simulink model "gm_rmsNormalization"  (R2025a)
settings: Solver=FixedStepDiscrete  StartTime=0.0  StopTime=simStopTime  FixedStep=1  RelTol=1e-3
libraries: simulink x23
(part 2 of 3)

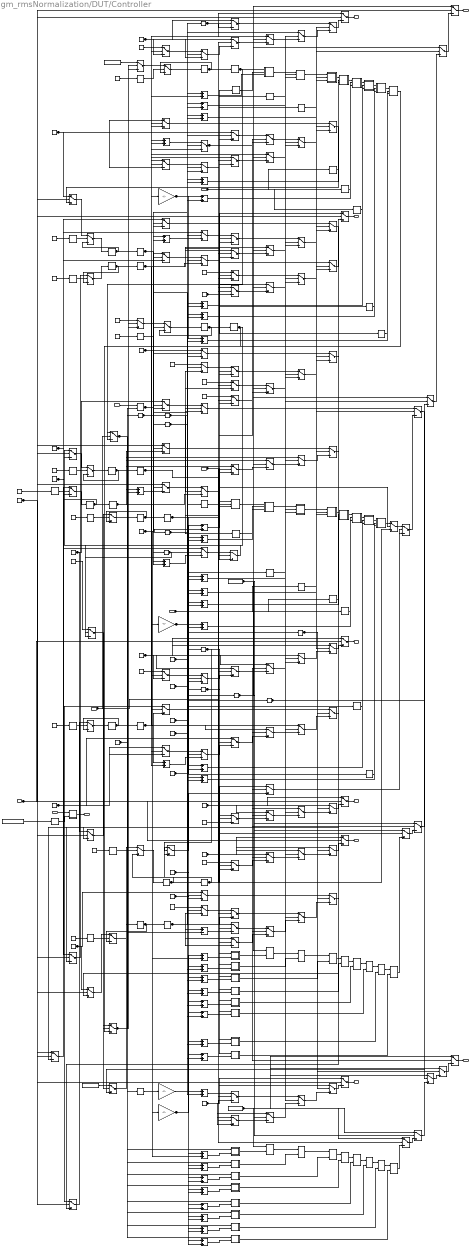
== system gm_rmsNormalization/DUT/Controller ==
  reset : Inport  OutDataTypeStr=boolean  PortDimensions=1  SampleTime=1
  start : Inport  Port=2  OutDataTypeStr=boolean  PortDimensions=1  SampleTime=1
  cfgGammaBeat : Inport  Port=3  OutDataTypeStr=single  PortDimensions=[1 8]  SampleTime=1
  cfgGammaValid : Inport  Port=4  OutDataTypeStr=boolean  PortDimensions=1  SampleTime=1
  ddrDataBeat : Inport  Port=5  OutDataTypeStr=single  PortDimensions=[1 8]  SampleTime=1
  ddrDataValid : Inport  Port=6  OutDataTypeStr=boolean  PortDimensions=1  SampleTime=1
  currentSumIn : Inport  Port=7  OutDataTypeStr=single  PortDimensions=1  SampleTime=1
  Assignment : Assignment  IndexOptions=Index vector (dialog)  Indices=double(8)  OutputSizes=double(0)
  Assignment1 : Assignment  IndexOptions=Index vector (dialog)  Indices=double(8)  OutputSizes=double(0)
  Assignment10 : Assignment  IndexOptions=Index vector (dialog)  Indices=double(3)  OutputSizes=double(0)
  Assignment11 : Assignment  IndexOptions=Index vector (dialog)  Indices=double(3)  OutputSizes=double(0)
  Assignment12 : Assignment  IndexOptions=Index vector (dialog)  Indices=double(2)  OutputSizes=double(0)
  Assignment13 : Assignment  IndexOptions=Index vector (dialog)  Indices=double(2)  OutputSizes=double(0)
  Assignment14 : Assignment  IndexOptions=Index vector (dialog)  Indices=double(1)  OutputSizes=double(0)
  Assignment15 : Assignment  IndexOptions=Index vector (dialog)  Indices=double(1)  OutputSizes=double(0)
  Assignment16 : Subsystem
  Assignment17 : Subsystem
  Assignment18 : Subsystem
  Assignment19 : Subsystem
  Assignment2 : Assignment  IndexOptions=Index vector (dialog)  Indices=double(7)  OutputSizes=double(0)
  Assignment20 : Subsystem
  Assignment21 : Subsystem
  Assignment22 : Subsystem
  Assignment23 : Subsystem
  Assignment24 : Subsystem
  Assignment25 : Subsystem
  Assignment26 : Subsystem
  Assignment27 : Subsystem
  Assignment28 : Subsystem
  Assignment29 : Subsystem
  Assignment3 : Assignment  IndexOptions=Index vector (dialog)  Indices=double(7)  OutputSizes=double(0)
  Assignment30 : Subsystem
  Assignment31 : Subsystem
  Assignment4 : Assignment  IndexOptions=Index vector (dialog)  Indices=double(6)  OutputSizes=double(0)
  Assignment5 : Assignment  IndexOptions=Index vector (dialog)  Indices=double(6)  OutputSizes=double(0)
  Assignment6 : Assignment  IndexOptions=Index vector (dialog)  Indices=double(5)  OutputSizes=double(0)
  Assignment7 : Assignment  IndexOptions=Index vector (dialog)  Indices=double(5)  OutputSizes=double(0)
  Assignment8 : Assignment  IndexOptions=Index vector (dialog)  Indices=double(4)  OutputSizes=double(0)
  Assignment9 : Assignment  IndexOptions=Index vector (dialog)  Indices=double(4)  OutputSizes=double(0)
  Selector : Subsystem
  Selector1 : Subsystem
  Selector10 : Selector  InputPortWidth=8  IndexOptions=Index vector (dialog)  Indices=double(7)  OutputSizes=double(0)
  Selector11 : Subsystem
  Selector12 : Subsystem
  Selector13 : Selector  InputPortWidth=8  IndexOptions=Index vector (dialog)  Indices=double(6)  OutputSizes=double(0)
  Selector14 : Subsystem
  Selector15 : Subsystem
  Selector16 : Selector  InputPortWidth=8  IndexOptions=Index vector (dialog)  Indices=double(5)  OutputSizes=double(0)
  Selector17 : Subsystem
  Selector18 : Subsystem
  Selector19 : Selector  InputPortWidth=8  IndexOptions=Index vector (dialog)  Indices=double(4)  OutputSizes=double(0)
  Selector2 : Subsystem
  Selector20 : Subsystem
  Selector21 : Selector  InputPortWidth=8  IndexOptions=Index vector (dialog)  Indices=double(8)  OutputSizes=double(0)
  Selector22 : Selector  InputPortWidth=8  IndexOptions=Index vector (dialog)  Indices=double(3)  OutputSizes=double(0)
  Selector23 : Selector  InputPortWidth=8  IndexOptions=Index vector (dialog)  Indices=double(7)  OutputSizes=double(0)
  Selector24 : Selector  InputPortWidth=8  IndexOptions=Index vector (dialog)  Indices=double(2)  OutputSizes=double(0)
  Selector25 : Selector  InputPortWidth=8  IndexOptions=Index vector (dialog)  Indices=double(6)  OutputSizes=double(0)
  Selector26 : Selector  InputPortWidth=8  IndexOptions=Index vector (dialog)  Indices=double(1)  OutputSizes=double(0)
  Selector27 : Selector  InputPortWidth=8  IndexOptions=Index vector (dialog)  Indices=double(5)  OutputSizes=double(0)
  Selector28 : Selector  InputPortWidth=8  IndexOptions=Index vector (dialog)  Indices=double(4)  OutputSizes=double(0)
  Selector29 : Selector  InputPortWidth=8  IndexOptions=Index vector (dialog)  Indices=double(3)  OutputSizes=double(0)
  Selector3 : Subsystem
  Selector30 : Selector  InputPortWidth=8  IndexOptions=Index vector (dialog)  Indices=double(2)  OutputSizes=double(0)
  Selector31 : Selector  InputPortWidth=8  IndexOptions=Index vector (dialog)  Indices=double(1)  OutputSizes=double(0)
  Selector4 : Subsystem
  Selector5 : Subsystem
  Selector6 : Subsystem
  Selector7 : Selector  InputPortWidth=8  IndexOptions=Index vector (dialog)  Indices=double(8)  OutputSizes=double(0)
  Selector8 : Subsystem
  Selector9 : Subsystem
  adder{,1..32,34..35,37..38} (37 alike) : Sum  OutDataTypeStr=uint16  AccumDataTypeStr=uint16  RndMeth=Nearest  SaturateOnIntegerOverflow=on  SampleTime=1
  adder33 : Subsystem
      mask Display: disp('NFP\nadd');
  adder36 : Sum  OutDataTypeStr=uint8  AccumDataTypeStr=uint8  RndMeth=Nearest  SaturateOnIntegerOverflow=on  SampleTime=1
  and : Logic  AllPortsSameDT=off  OutDataTypeStr=boolean  SampleTime=1
  compare : simulink/Logic and Bit Operations/Compare To Constant  relop=~=  const=0  OutDataTypeStr=boolean
  compare1 : simulink/Logic and Bit Operations/Compare To Constant  relop===  const=191  OutDataTypeStr=boolean
  compare10 : simulink/Logic and Bit Operations/Compare To Constant  relop=<  const=192  OutDataTypeStr=boolean
  compare2 : simulink/Logic and Bit Operations/Compare To Constant  relop===  const=63  OutDataTypeStr=boolean
  compare3 : simulink/Logic and Bit Operations/Compare To Constant  relop===  const=3  OutDataTypeStr=boolean
  compare4 : simulink/Logic and Bit Operations/Compare To Constant  relop===  const=1  OutDataTypeStr=boolean
  compare5 : simulink/Logic and Bit Operations/Compare To Constant  relop===  const=191  OutDataTypeStr=boolean
  compare6 : simulink/Logic and Bit Operations/Compare To Constant  relop===  const=0  OutDataTypeStr=boolean
  compare7 : simulink/Logic and Bit Operations/Compare To Constant  relop===  const=191  OutDataTypeStr=boolean
  compare8 : simulink/Logic and Bit Operations/Compare To Constant  relop===  const=2  OutDataTypeStr=boolean
  compare9 : simulink/Logic and Bit Operations/Compare To Constant  relop===  const=0  OutDataTypeStr=boolean
  const : Constant  Value=single(0.0015360000543296337)  VectorParams1D=off  OutDataTypeStr=single  SampleTime=1
  const1 : Constant  Value="repmat(single(0),[1  8])"  VectorParams1D=off  OutDataTypeStr=single  SampleTime=1
  const{8..11,13..14} (6 alike) : Constant  VectorParams1D=off  OutDataTypeStr=boolean  SampleTime=1
  const12 : Constant  Value=0  VectorParams1D=off  OutDataTypeStr=uint8  SampleTime=1
  const{3..4,6..7,15,19} (6 alike) : Constant  Value=0  VectorParams1D=off  OutDataTypeStr=boolean  SampleTime=1
  const16 : Constant  VectorParams1D=off  OutDataTypeStr=uint8  SampleTime=1
  const17 : Constant  Value=8  VectorParams1D=off  OutDataTypeStr=uint16  SampleTime=1
  const{5,18,27..28,35} (5 alike) : Constant  Value=0  VectorParams1D=off  OutDataTypeStr=uint16  SampleTime=1
  const2 : Constant  Value="repmat(single(0),[1  8])"  VectorParams1D=off  OutDataTypeStr=single  SampleTime=1
  const20 : Constant  Value=7  VectorParams1D=off  OutDataTypeStr=uint16  SampleTime=1
  const21 : Constant  Value=4  VectorParams1D=off  OutDataTypeStr=uint8  SampleTime=1
  const22 : Constant  Value=3  VectorParams1D=off  OutDataTypeStr=uint8  SampleTime=1
  const23 : Constant  Value=2  VectorParams1D=off  OutDataTypeStr=uint8  SampleTime=1
  const24 : Constant  Value="repmat(single(0),[1  1536])"  VectorParams1D=off  OutDataTypeStr=single  SampleTime=1
  const25 : Constant  Value=6  VectorParams1D=off  OutDataTypeStr=uint16  SampleTime=1
  const26 : Constant  Value=0  VectorParams1D=off  OutDataTypeStr=uint8  SampleTime=1
  const29 : Constant  Value=5  VectorParams1D=off  OutDataTypeStr=uint16  SampleTime=1
  const30 : Constant  Value="repmat(single(0),[1  1536])"  VectorParams1D=off  OutDataTypeStr=single  SampleTime=1
  const31 : Constant  Value=4  VectorParams1D=off  OutDataTypeStr=uint16  SampleTime=1
  const32 : Constant  Value=3  VectorParams1D=off  OutDataTypeStr=uint16  SampleTime=1
  const33 : Constant  VectorParams1D=off  OutDataTypeStr=uint16  SampleTime=1
  const34 : Constant  Value=0  VectorParams1D=off  OutDataTypeStr=uint8  SampleTime=1
  const36 : Constant  Value=2  VectorParams1D=off  OutDataTypeStr=uint16  SampleTime=1
  const37 : Constant  VectorParams1D=off  OutDataTypeStr=uint8  SampleTime=1
  const38 : Constant  Value=22  VectorParams1D=off  OutDataTypeStr=uint8  SampleTime=1
  delayMatch : Delay  DelayLength=double(70)  InitialCondition=0  SampleTime=1
  delayMatch{1..10} (10 alike) : Delay  DelayLength=double(41)  InitialCondition=0  SampleTime=1
  dtc : DataTypeConversion  OutDataTypeStr=uint16  RndMeth=Nearest  SampleTime=1
  gain : Gain  Gain="fi(0,0,16,0,\"hex\",\"00c0\")"  ParamDataTypeStr=fixdt(0, 16, 0)  OutDataTypeStr=uint16  RndMeth=Nearest  SaturateOnIntegerOverflow=on  SampleTime=1
  gain1 : Gain  Gain="fi(0,0,16,0,\"hex\",\"0008\")"  ParamDataTypeStr=fixdt(0, 16, 0)  OutDataTypeStr=uint16  RndMeth=Nearest  SaturateOnIntegerOverflow=on  SampleTime=1
  gain2 : Gain  Gain="fi(0,0,16,0,\"hex\",\"0008\")"  ParamDataTypeStr=fixdt(0, 16, 0)  OutDataTypeStr=uint16  RndMeth=Nearest  SaturateOnIntegerOverflow=on  SampleTime=1
  gain3 : Gain  Gain="fi(0,0,16,0,\"hex\",\"0008\")"  ParamDataTypeStr=fixdt(0, 16, 0)  OutDataTypeStr=uint16  RndMeth=Nearest  SaturateOnIntegerOverflow=on  SampleTime=1
  intdelay{,1..9} (10 alike) : Delay  DelayLength=double(1)  InitialCondition=0  SampleTime=1
  intdelay_enbsw{,4,6,9} (4 alike) : Switch  Criteria=u2 ~= 0  Threshold=double(0)  OutDataTypeStr=uint16  SampleTime=1  SaturateOnIntegerOverflow=off  InputSameDT=off
  intdelay_enbsw1 : Switch  Criteria=u2 ~= 0  Threshold=double(0)  OutDataTypeStr=boolean  SampleTime=1  SaturateOnIntegerOverflow=off  InputSameDT=off
  intdelay_enbsw2 : Switch  Criteria=u2 ~= 0  Threshold=double(0)  OutDataTypeStr=uint8  SampleTime=1  SaturateOnIntegerOverflow=off  InputSameDT=off
  intdelay_enbsw3 : Switch  Criteria=u2 ~= 0  Threshold=double(0)  OutDataTypeStr=uint8  SampleTime=1  SaturateOnIntegerOverflow=off  InputSameDT=off
  intdelay_enbsw5 : Switch  Criteria=u2 ~= 0  Threshold=double(0)  OutDataTypeStr=uint8  SampleTime=1  SaturateOnIntegerOverflow=off  InputSameDT=off
  intdelay_enbsw7 : Switch  Criteria=u2 ~= 0  Threshold=double(0)  OutDataTypeStr=single  SampleTime=1  SaturateOnIntegerOverflow=off  InputSameDT=off
  intdelay_enbsw8 : Switch  Criteria=u2 ~= 0  Threshold=double(0)  OutDataTypeStr=single  SampleTime=1  SaturateOnIntegerOverflow=off  InputSameDT=off
  sigspec{,2,5,9} (4 alike) : SignalSpecification  OutDataTypeStr=uint16  Dimensions=1
  sigspec1 : SignalSpecification  OutDataTypeStr=boolean  Dimensions=1
  sigspec3 : SignalSpecification  OutDataTypeStr=uint8  Dimensions=1
  sigspec4 : SignalSpecification  OutDataTypeStr=uint8  Dimensions=1
  sigspec6 : SignalSpecification  OutDataTypeStr=uint8  Dimensions=1
  sigspec7 : SignalSpecification  OutDataTypeStr=single  Dimensions=[1, 1536]
  sigspec8 : SignalSpecification  OutDataTypeStr=single  Dimensions=[1, 1536]
  stateControl{,1..9} (10 alike) : Constant  OutDataTypeStr=boolean  SampleTime=1
  subtract : Sum  Inputs=+-  OutDataTypeStr=uint8  AccumDataTypeStr=uint8  RndMeth=Nearest  SaturateOnIntegerOverflow=on  SampleTime=1
  switch{,1,8..9,16..17,25..26,35..36,99..106} (18 alike) : Switch  Criteria=u2 ~= 0  Threshold="fi(0,0,1,0,\"hex\",\"0\")"  OutDataTypeStr=single  SampleTime=1  SaturateOnIntegerOverflow=off  InputSameDT=off
  switch{2..3,5..7,10..11,13..15,18..19,21..24,27..28,31..34,37..38,40..46,50..52} (34 alike) : Switch  Criteria=u2 ~= 0  Threshold="fi(0,0,1,0,\"hex\",\"0\")"  OutDataTypeStr=boolean  SampleTime=1  SaturateOnIntegerOverflow=off  InputSameDT=off
  switch{4,12,20,29..30,39,47..49,53..58,74,82..90,97..98,107..117} (38 alike) : Switch  Criteria=u2 ~= 0  Threshold="fi(0,0,1,0,\"hex\",\"0\")"  OutDataTypeStr=uint16  SampleTime=1  SaturateOnIntegerOverflow=off  InputSameDT=off
  switch{59..73,75..81,91..96} (28 alike) : Switch  Criteria=u2 ~= 0  Threshold="fi(0,0,1,0,\"hex\",\"0\")"  OutDataTypeStr=uint8  SampleTime=1  SaturateOnIntegerOverflow=off  InputSameDT=off
  rsqrtOperand : Outport  SampleTime=1
  xBeatOut : Outport  Port=2  SampleTime=1
  gBeatOut : Outport  Port=3  SampleTime=1
  captureInvRms : Outport  Port=4  SampleTime=1
  outValid : Outport  Port=5  SampleTime=1
  ddrReadAddr : Outport  Port=6  SampleTime=1
  ddrReadEn : Outport  Port=7  SampleTime=1
  done : Outport  Port=8  SampleTime=1
  busy : Outport  Port=9  SampleTime=1
  wires:
  switch31/1 -> switch21/3
  intdelay_enbsw8/1 -> intdelay8/1
  const15/1 -> switch46/1
  Assignment26/1(Out1) -> Assignment27/1(In1)
  Assignment29/1(Out1) -> Assignment30/1(In1)
  Assignment1/1 -> switch36/3
  switch41/1 -> switch33/3
  switch34/1 -> switch23/3
  switch9/1 -> switch1/3
  Selector29/1 -> Assignment18/2(In2)
  switch104/1 -> intdelay_enbsw7/1
  Assignment24/1(Out1) -> Assignment25/1(In1)
  const30/1 -> switch105/1
  adder26/1 -> Assignment21/3(In3)
  Assignment13/1 -> Assignment11/1
  Assignment8/1 -> Assignment6/1
  Assignment21/1(Out1) -> Assignment22/1(In1)
  switch52/1 -> switch51/1
  switch39/1 -> switch29/3
  switch66/1 -> switch67/1
  switch14/1 -> switch6/3
  Selector4/1(Out1) -> Assignment4/2
  switch42/1 -> switch34/3
  switch25/1 -> switch16/3
  switch27/1 -> switch18/3
  switch10/1 -> switch2/3
  delayMatch10/1 -> intdelay_enbsw4/2
  switch12/1 -> switch4/3
  switch46/1 -> switch44/1
  Selector30/1 -> Assignment17/2(In2)
  adder2/1 -> Selector1/2(In2)
  switch15/1 -> switch7/3
  switch22/1 -> switch14/3
  switch60/1 -> switch61/3
  const10/1 -> switch37/1
  Assignment7/1 -> Assignment5/1
  const19/1 -> switch50/1
  compare6/1 -> switch65/2, switch72/2
  switch18/1 -> switch10/3
  const9/1 -> switch32/1
  adder25/1 -> Assignment25/3(In3)
  Assignment10/1 -> Assignment8/1
  adder10/1 -> Selector8/2(In2)
  switch72/1 -> switch62/1
  Assignment11/1 -> Assignment9/1
  switch65/1 -> switch64/1
  delayMatch6/1 -> intdelay_enbsw6/2
  switch101/1 -> switch102/1
  adder14/1 -> Selector12/2(In2)
  switch1/1 -> gBeatOut/1
  switch53/1 -> switch55/3
  switch51/1 -> switch50/3, and/2
  const23/1 -> switch91/1
  const36/1 -> adder25/2, adder31/2, adder17/2, adder19/2
  adder38/1 -> switch111/1
  switch28/1 -> switch19/3
  switch33/1 -> switch22/3
  delayMatch2/1 -> intdelay_enbsw9/2
  Selector26/1 -> Assignment24/2(In2)
  compare2/1 -> switch82/2, switch107/2, switch45/2, switch59/2, switch46/2, switch54/2, switch75/2
  currentSumIn/1 -> adder33/1(In1)
  switch87/1 -> switch89/3
  Selector19/1 -> Assignment27/2(In2)
  sigspec/1 -> gain2/1, compare1/1, adder34/1, switch48/3
  switch85/1 -> switch86/1
  switch40/1 -> switch31/3
  gain1/1 -> adder13/1, adder7/1, adder1/1, adder8/1, adder11/1, adder4/1, adder3/1, adder21/1, adder10/1, adder16/1, adder19/1, adder5/1, adder14/1, adder17/1, adder23/1, adder2/1
  switch23/1 -> switch15/3
  sigspec1/1 -> switch52/3, switch51/3
  const35/1 -> switch90/1, switch85/1, switch82/3, switch88/1
  switch113/1 -> switch114/1
  intdelay_enbsw1/1 -> intdelay1/1
  switch/1 -> xBeatOut/1
  stateControl3/1 -> delayMatch4/1
  compare9/1 -> switch115/2, switch12/2, switch15/2, switch13/2, switch11/2, switch89/2, switch58/2, switch79/2, switch10/2, switch69/2, switch14/2, switch94/2, switch8/2, switch103/2, switch9/2
  Assignment17/1(Out1) -> Assignment18/1(In1)
  const29/1 -> adder28/2, adder8/2, adder15/2, adder10/2
  const20/1 -> adder3/2, adder4/2, adder9/2, adder24/2
  switch24/1 -> switch15/1
  switch74/1 -> switch83/3
  Assignment/1 -> switch35/3
  Selector9/1(Out1) -> Assignment8/2
  switch77/1 -> switch78/3
  adder13/1 -> Selector11/2(In2)
  const/1 -> delayMatch/1
  Selector3/1(Out1) -> Assignment3/2
  adder6/1 -> Assignment31/3(In3)
  adder31/1 -> Assignment17/3(In3)
  switch88/1 -> switch89/1
  sigspec2/1 -> gain1/1, compare7/1, adder35/1, switch97/3, switch57/1, switch56/1
  stateControl7/1 -> delayMatch8/1
  adder15/1 -> Assignment28/3(In3)
  const37/1 -> adder36/2, subtract/2
  const17/1 -> adder2/2, adder6/2, adder1/2, adder20/2
  switch70/1 -> switch69/1
  switch83/1 -> switch84/3
  const5/1 -> switch39/1, switch39/3, switch4/1, switch30/3, switch29/1, switch12/1
  Selector12/1(Out1) -> Assignment10/2
  Selector/1(Out1) -> Assignment/2
  adder20/1 -> Assignment23/3(In3)
  switch57/1 -> switch58/3
  stateControl1/1 -> delayMatch2/1
  cfgGammaValid/1 -> switch51/2, switch106/2, switch48/2
  intdelay_enbsw9/1 -> intdelay9/1
  compare10/1 -> switch111/2, switch32/2, switch30/2
  switch38/1 -> switch28/3
  compare1/1 -> switch47/2, switch52/2
  adder9/1 -> Assignment30/3(In3)
  Assignment12/1 -> Assignment10/1
  compare5/1 -> switch85/2, switch91/2, switch66/2, switch112/2
  compare7/1 -> switch44/2, switch53/2, switch43/2, switch108/2, switch60/2, switch73/2, switch74/2
  switch106/1 -> Selector11/1(In1), switch105/3, Selector5/1(In1), Selector1/1(In1), Selector14/1(In1), Selector20/1(In1), Selector8/1(In1), Selector17/1(In1), Selector3/1(In1)
  const26/1 -> switch81/1, switch80/1, switch75/1
  switch11/1 -> switch3/3
  intdelay2/1 -> sigspec3/1, intdelay_enbsw2/3
  switch78/1 -> switch79/3
  ddrDataBeat/1 -> Selector31/1, Selector27/1, Selector23/1, Selector28/1, Selector29/1, Selector30/1, Selector25/1, Selector21/1
  switch80/1 -> switch79/1
  stateControl6/1 -> delayMatch7/1
  intdelay4/1 -> sigspec5/1, intdelay_enbsw4/3
  Selector27/1 -> Assignment20/2(In2)
  sigspec3/1 -> compare6/1, subtract/1, switch70/3, switch66/3, switch63/3, switch63/1, switch65/1, switch67/3
  switch29/1 -> switch20/3
  Selector5/1(Out1) -> Assignment5/2
  switch108/1 -> switch109/3
  switch94/1 -> switch96/3
  const25/1 -> adder5/2, adder7/2, adder26/2, adder12/2
  switch116/1 -> switch115/1
  switch69/1 -> switch71/3
  const6/1 -> switch32/3, switch13/1, switch40/3, switch40/1, switch5/1, switch31/1
  Assignment31/1(Out1) -> switch106/1
  start/1 -> and/1
  sigspec5/1 -> gain3/1, switch82/1, switch88/3, adder37/1, compare5/1, switch83/1, switch74/3, switch86/3, switch84/1
  switch48/1 -> switch49/3
  switch84/1 -> switch87/3
  switch64/1 -> switch68/3
  gain3/1 -> adder30/1, adder26/1, adder31/1, adder20/1, adder24/1, adder28/1, adder29/1, adder32/1
  const7/1 -> switch14/1, switch45/3, switch22/1, switch43/3, switch33/1, switch41/1, switch6/1
  compare8/1 -> switch33/2, switch64/2, switch84/2, switch27/2, switch28/2, switch56/2, switch31/2, switch100/2, switch110/2, switch77/2, switch62/2, switch29/2, switch34/2, switch25/2, switch26/2
  switch4/1 -> ddrReadAddr/1
  adder7/1 -> Selector5/2(In2)
  switch99/1 -> switch100/3
  adder28/1 -> Assignment20/3(In3)
  Selector6/1(Out1) -> Assignment6/2
  sigspec7/1 -> Selector12/1(In1), Selector4/1(In1), Assignment16/1(In1), Selector18/1(In1), Selector/1(In1), Selector2/1(In1), Selector9/1(In1), Selector6/1(In1), Selector15/1(In1), switch103/1, switch100/1, switch101/3, switch99/1, switch99/3
  intdelay7/1 -> sigspec7/1, intdelay_enbsw7/3
  switch79/1 -> switch81/3
  switch98/1 -> intdelay_enbsw6/1
  adder30/1 -> Assignment18/3(In3)
  Selector23/1 -> Assignment22/2(In2)
  compare3/1 -> switch63/2, switch76/2, switch40/2, switch109/2, switch61/2, switch42/2, switch38/2, switch39/2, switch37/2, switch41/2, switch55/2, switch83/2, switch35/2, switch36/2, switch99/2
  adder29/1 -> Assignment19/3(In3)
  switch45/1 -> switch43/1
  switch86/1 -> switch87/1
  Assignment28/1(Out1) -> Assignment29/1(In1)
  intdelay1/1 -> sigspec1/1, intdelay_enbsw1/3
  intdelay/1 -> sigspec/1, intdelay_enbsw/3
  switch117/1 -> intdelay_enbsw9/1
  sigspec6/1 -> switch60/3, compare3/1, compare/1, switch91/3, switch95/3, compare4/1, compare8/1, switch92/3, switch72/3, compare9/1
  const21/1 -> switch61/1
  switch76/1 -> switch77/3
  switch58/1 -> switch98/3
  const4/1 -> switch38/1, switch11/1, switch3/1, switch28/1, switch19/1
  switch67/1 -> switch68/1
  stateControl2/1 -> delayMatch3/1
  adder19/1 -> Selector17/2(In2)
  compare4/1 -> switch93/2, switch23/2, switch57/2, switch21/2, switch78/2, switch87/2, switch22/2, switch114/2, switch68/2, switch18/2, switch19/2, switch20/2, switch16/2, switch102/2, switch17/2
  Selector8/1(Out1) -> Assignment7/2
  intdelay8/1 -> sigspec8/1, intdelay_enbsw8/3
  switch100/1 -> switch102/3
  Assignment6/1 -> Assignment4/1
  const16/1 -> switch59/3, switch95/1
  Selector31/1 -> Assignment16/2(In2)
  switch89/1 -> switch90/3
  switch16/1 -> switch8/3
  Selector11/1(Out1) -> Assignment9/2
  sigspec4/1 -> adder36/1, dtc/1, compare2/1, switch80/3, switch77/1, switch78/1, switch73/3, switch76/1
  intdelay_enbsw/1 -> intdelay/1
  sigspec9/1 -> switch108/3, switch116/3, compare10/1, adder38/1, switch107/1, adder/2, switch109/1, switch111/3, switch110/1
  switch47/1 -> switch48/1
  const8/1 -> switch46/3, switch34/1, switch24/1, switch44/3, switch42/1, switch23/1
  switch21/1 -> switch13/3
  switch112/1 -> switch113/1
  switch103/1 -> switch104/3
  ddrDataValid/1 -> switch86/2, switch92/2, switch67/2, switch101/2, switch113/2
  Selector25/1 -> Assignment21/2(In2)
  delayMatch/1 -> adder33/2(In2)
  const3/1 -> switch37/3, switch18/1, switch10/1, switch27/1, switch2/1
  Selector15/1(Out1) -> Assignment12/2
  const2/1 -> Assignment15/1, switch26/1, switch17/1, switch9/1, switch36/1, switch1/1
  const27/1 -> switch98/1, switch54/1, switch97/1, switch55/1, switch54/3
  intdelay9/1 -> sigspec9/1, intdelay_enbsw9/3
  compare/1 -> switch24/3, switch7/1
  adder/1 -> switch30/1
  Selector16/1 -> Assignment28/2(In2)
  intdelay_enbsw6/1 -> intdelay6/1
  adder33/1(Out1) -> rsqrtOperand/1
  Selector7/1 -> Assignment31/2(In2)
  const18/1 -> switch117/1, switch116/1, switch112/1, switch107/3
  Assignment27/1(Out1) -> Assignment28/1(In1)
  intdelay_enbsw2/1 -> intdelay2/1
  reset/1 -> switch81/2, switch71/2, switch4/2, switch6/2, switch5/2, switch105/2, switch104/2, switch90/2, switch50/2, switch1/2, switch/2, switch98/2, switch7/2, switch3/2, switch117/2, switch2/2, switch96/2, switch49/2
  Selector2/1(Out1) -> Assignment2/2
  Selector28/1 -> Assignment19/2(In2)
  intdelay3/1 -> intdelay_enbsw3/3, sigspec4/1
  switch96/1 -> intdelay_enbsw5/1
  adder37/1 -> switch85/3
  adder24/1 -> Assignment22/3(In3)
  Assignment23/1(Out1) -> switch101/1
  and/1 -> switch97/2, switch80/2, switch88/2, switch116/2, switch24/2, switch70/2, switch95/2
  Selector13/1 -> Assignment29/2(In2)
  intdelay_enbsw4/1 -> intdelay4/1
  const32/1 -> adder22/2, adder14/2, adder16/2, adder30/2
  const34/1 -> switch70/1, switch71/1
  switch92/1 -> switch93/1
  switch55/1 -> switch56/3
  intdelay5/1 -> sigspec6/1, intdelay_enbsw5/3
  switch111/1 -> switch112/3, switch113/3
  const1/1 -> Assignment14/1, switch8/1, switch35/1, switch16/1, switch25/1, switch/1
  stateControl/1 -> delayMatch1/1
  switch30/1 -> switch20/1
  switch6/1 -> done/1
  switch7/1 -> busy/1
  Assignment5/1 -> Assignment3/1
  adder16/1 -> Selector14/2(In2)
  intdelay_enbsw3/1 -> intdelay3/1
  stateControl9/1 -> delayMatch10/1
  const28/1 -> switch49/1, switch47/1
  switch73/1 -> switch76/3
  cfgGammaBeat/1 -> Selector26/1, Selector16/1, Selector24/1, Selector13/1, Selector7/1, Selector22/1, Selector19/1, Selector10/1
  adder21/1 -> Selector18/2(In2)
  switch37/1 -> switch27/3
  adder36/1 -> switch75/3
  switch2/1 -> captureInvRms/1
  switch36/1 -> switch26/3
  switch20/1 -> switch12/3
  Selector10/1 -> Assignment30/2(In2)
  intdelay_enbsw5/1 -> intdelay5/1
  Selector1/1(Out1) -> Assignment1/2
  switch82/1 -> switch74/1
  Selector24/1 -> Assignment25/2(In2)
  adder23/1 -> Selector20/2(In2)
  const11/1 -> switch38/3
  switch107/1 -> switch108/1
  switch59/1 -> switch60/1
  const38/1 -> switch66/1
  delayMatch3/1 -> intdelay_enbsw1/2
  switch50/1 -> intdelay_enbsw1/1
  switch75/1 -> switch73/1
  delayMatch7/1 -> intdelay_enbsw/2
  Assignment18/1(Out1) -> Assignment19/1(In1)
  Assignment3/1 -> Assignment1/1
  switch68/1 -> switch69/3
  gain2/1 -> adder9/1, adder18/1, adder12/1, adder22/1, adder6/1, adder25/1, adder27/1, adder15/1
  const24/1 -> switch104/1
  Assignment19/1(Out1) -> Assignment20/1(In1)
  const31/1 -> adder18/2, adder29/2, adder13/2, adder11/2
  stateControl5/1 -> delayMatch6/1
  delayMatch8/1 -> intdelay_enbsw8/2
  Assignment20/1(Out1) -> Assignment21/1(In1)
  switch35/1 -> switch25/3
  switch17/1 -> switch9/3
  Assignment15/1 -> Assignment13/1
  switch13/1 -> switch5/3
  switch26/1 -> switch17/3
  stateControl8/1 -> delayMatch9/1
  Assignment22/1(Out1) -> Assignment23/1(In1)
  switch102/1 -> switch103/3
  switch115/1 -> switch117/3
  adder27/1 -> Assignment24/3(In3)
  gain/1 -> adder/1
  switch8/1 -> switch/3
  Selector22/1 -> Assignment26/2(In2)
  switch90/1 -> intdelay_enbsw4/1
  Assignment30/1(Out1) -> Assignment31/1(In1)
  switch109/1 -> switch110/3
  switch93/1 -> switch94/3
  switch61/1 -> switch62/3
  Selector21/1 -> Assignment23/2(In2)
  switch110/1 -> switch114/3
  adder18/1 -> Assignment27/3(In3)
  const14/1 -> switch45/1
  switch32/1 -> switch21/1
  const33/1 -> adder34/2, adder38/2, adder35/2, adder37/2, adder32/2, adder27/2, adder21/2, adder23/2
  stateControl4/1 -> delayMatch5/1
  switch62/1 -> switch93/3
  Assignment25/1(Out1) -> Assignment26/1(In1)
  switch95/1 -> switch94/1
  adder12/1 -> Assignment29/3(In3)
  Assignment4/1 -> Assignment2/1
  switch5/1 -> ddrReadEn/1
  const12/1 -> switch96/1, switch59/1
  switch56/1 -> switch57/3
  Assignment9/1 -> Assignment7/1
  Selector18/1(Out1) -> Assignment14/2
  switch71/1 -> intdelay_enbsw2/1
  Selector17/1(Out1) -> Assignment13/2
  switch44/1 -> switch42/3
  adder34/1 -> switch47/3
  delayMatch9/1 -> intdelay_enbsw2/2
  switch49/1 -> intdelay_enbsw/1
  Selector14/1(Out1) -> Assignment11/2
  adder35/1 -> switch53/3
  switch105/1 -> intdelay_enbsw8/1
  switch97/1 -> switch58/1
  switch81/1 -> intdelay_enbsw3/1
  intdelay_enbsw7/1 -> intdelay7/1
  switch19/1 -> switch11/3
  adder5/1 -> Selector4/2(In2)
  switch3/1 -> outValid/1
  Assignment16/1(Out1) -> Assignment17/1(In1)
  subtract/1 -> switch65/3
  switch91/1 -> switch92/1
  switch114/1 -> switch115/3
  delayMatch5/1 -> intdelay_enbsw3/2
  intdelay6/1 -> sigspec2/1, intdelay_enbsw6/3
  adder22/1 -> Assignment26/3(In3)
  Assignment2/1 -> Assignment/1
  adder8/1 -> Selector6/2(In2)
  const22/1 -> switch72/1
  adder11/1 -> Selector9/2(In2)
  adder17/1 -> Selector15/2(In2)
  delayMatch4/1 -> intdelay_enbsw7/2
  switch43/1 -> switch41/3
  adder4/1 -> Selector3/2(In2)
  adder3/1 -> Selector2/2(In2)
  dtc/1 -> gain/1
  Selector20/1(Out1) -> Assignment15/2
  switch63/1 -> switch64/3
  adder32/1 -> Assignment16/3(In3)
  sigspec8/1 -> Assignment24/1(In1), switch106/3
  switch54/1 -> switch53/1
  const13/1 -> switch52/1
  delayMatch1/1 -> intdelay_enbsw5/2
  adder1/1 -> Selector/2(In2)
  Assignment14/1 -> Assignment12/1

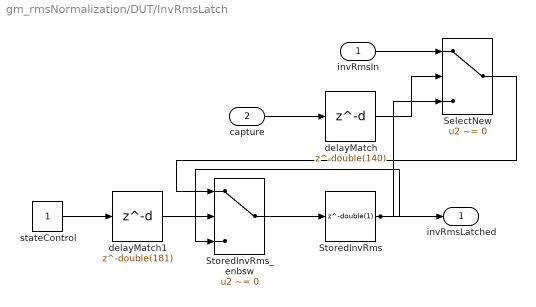
== system gm_rmsNormalization/DUT/InvRmsLatch ==
  invRmsIn : Inport  OutDataTypeStr=single  PortDimensions=1  SampleTime=1
  capture : Inport  Port=2  OutDataTypeStr=boolean  PortDimensions=1  SampleTime=1
  SelectNew : Switch  Criteria=u2 ~= 0  Threshold="fi(0,0,1,0,\"hex\",\"0\")"  OutDataTypeStr=single  SampleTime=1  SaturateOnIntegerOverflow=off  InputSameDT=off
  StoredInvRms : Delay  DelayLength=double(1)  InitialCondition=0  SampleTime=1
  StoredInvRms_enbsw : Switch  Criteria=u2 ~= 0  Threshold=double(0)  OutDataTypeStr=single  SampleTime=1  SaturateOnIntegerOverflow=off  InputSameDT=off
  delayMatch : Delay  DelayLength=double(140)  InitialCondition=0  SampleTime=1
  delayMatch1 : Delay  DelayLength=double(181)  InitialCondition=0  SampleTime=1
  stateControl : Constant  OutDataTypeStr=boolean  SampleTime=1
  invRmsLatched : Outport  SampleTime=1
  wires:
  delayMatch/1 -> SelectNew/2
  invRmsIn/1 -> SelectNew/1
  SelectNew/1 -> StoredInvRms_enbsw/1
  capture/1 -> delayMatch/1
  StoredInvRms/1 -> invRmsLatched/1, StoredInvRms_enbsw/3, SelectNew/3
  StoredInvRms_enbsw/1 -> StoredInvRms/1
  delayMatch1/1 -> StoredInvRms_enbsw/2
  stateControl/1 -> delayMatch1/1

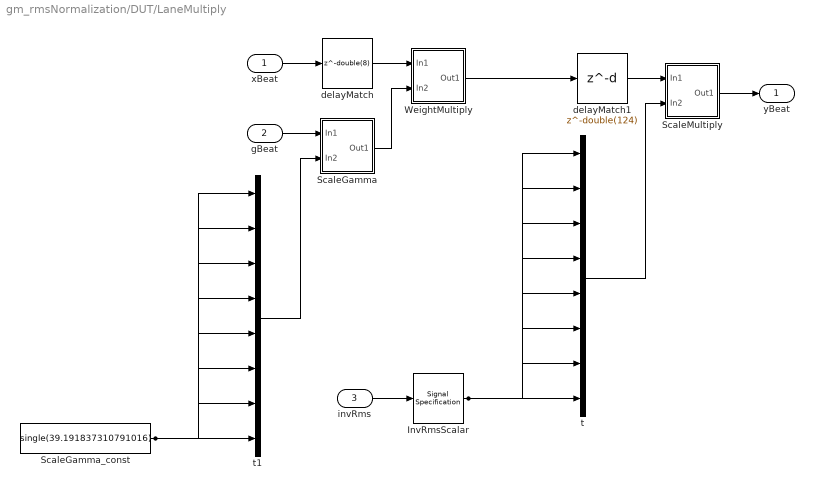
== system gm_rmsNormalization/DUT/LaneMultiply ==
  xBeat : Inport  OutDataTypeStr=single  PortDimensions=[1 8]  SampleTime=1
  gBeat : Inport  Port=2  OutDataTypeStr=single  PortDimensions=[1 8]  SampleTime=1
  invRms : Inport  Port=3  OutDataTypeStr=single  PortDimensions=1  SampleTime=1
  InvRmsScalar : SignalSpecification  OutDataTypeStr=single  Dimensions=1
  ScaleGamma : Subsystem
      mask Display: disp('NFP\nmul');
  ScaleGamma_const : Constant  Value=single(39.191837310791016)  OutDataTypeStr=single  SampleTime=1
  ScaleMultiply : Subsystem
      mask Display: disp('NFP\nmul');
  WeightMultiply : Subsystem
      mask Display: disp('NFP\nmul');
  delayMatch : Delay  DelayLength=double(8)  InitialCondition=0  SampleTime=1
  delayMatch1 : Delay  DelayLength=double(124)  InitialCondition=0  SampleTime=1
  t : Mux  Inputs=8
  t1 : Mux  Inputs=8
  yBeat : Outport  SampleTime=1
  wires:
  ScaleMultiply/1(Out1) -> yBeat/1
  t/1 -> ScaleMultiply/2(In2)
  WeightMultiply/1(Out1) -> delayMatch1/1
  delayMatch1/1 -> ScaleMultiply/1(In1)
  delayMatch/1 -> WeightMultiply/1(In1)
  invRms/1 -> InvRmsScalar/1
  t1/1 -> ScaleGamma/2(In2)
  InvRmsScalar/1 -> t/1, t/2, t/3, t/5, t/4, t/6, t/7, t/8
  gBeat/1 -> ScaleGamma/1(In1)
  xBeat/1 -> delayMatch/1
  ScaleGamma/1(Out1) -> WeightMultiply/2(In2)
  ScaleGamma_const/1 -> t1/1, t1/2, t1/3, t1/5, t1/4, t1/6, t1/7, t1/8

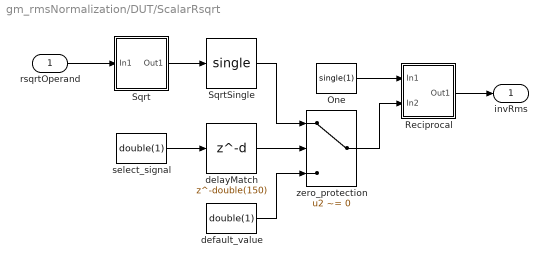
== system gm_rmsNormalization/DUT/ScalarRsqrt ==
  rsqrtOperand : Inport  OutDataTypeStr=single  PortDimensions=1  SampleTime=1
  One : Constant  Value=single(1)  OutDataTypeStr=single  SampleTime=1
  Reciprocal : Subsystem
      mask Display: disp('NFP\nmul');
  Sqrt : Subsystem
      mask Display: disp('NFP\nsqrt');
  SqrtSingle : DataTypeConversion  OutDataTypeStr=single
  default_value : Constant  Value=double(1)  OutDataTypeStr=single  SampleTime=1
  delayMatch : Delay  DelayLength=double(150)  InitialCondition=0  SampleTime=1
  select_signal : Constant  Value=double(1)  OutDataTypeStr=boolean  SampleTime=1
  zero_protection : Switch  Criteria=u2 ~= 0  Threshold=double(0)  OutDataTypeStr=single  SampleTime=1  SaturateOnIntegerOverflow=off  InputSameDT=off
  invRms : Outport  SampleTime=1
  wires:
  Reciprocal/1(Out1) -> invRms/1
  One/1 -> Reciprocal/1(In1)
  default_value/1 -> zero_protection/3
  delayMatch/1 -> zero_protection/2
  SqrtSingle/1 -> zero_protection/1
  zero_protection/1 -> Reciprocal/2(In2)
  select_signal/1 -> delayMatch/1
  Sqrt/1(Out1) -> SqrtSingle/1
  rsqrtOperand/1 -> Sqrt/1(In1)

== system gm_rmsNormalization/DUT/SquareBeat ==
  ddrDataBeat : Inport  OutDataTypeStr=single  PortDimensions=[8]  SampleTime=1
  Square : Subsystem
      mask Display: disp('NFP\nmul');
  squaredBeat : Outport  SampleTime=1
  wires:
  Square/1(Out1) -> squaredBeat/1
  ddrDataBeat/1 -> Square/1(In1), Square/2(In2)

== system gm_rmsNormalization/DUT/BeatAccumulator/AccumulateAdd00 ==
  In1 : Inport
  In2 : Inport  Port=2
  AccumulateAdd00 : Sum  OutDataTypeStr=single  SampleTime=1
  AccumulateAdd00_pd1 : Delay  DelayLength=11
  Out1 : Outport
  wires:
  In1/1 -> AccumulateAdd00/1
  In2/1 -> AccumulateAdd00/2
  AccumulateAdd00/1 -> AccumulateAdd00_pd1/1
  AccumulateAdd00_pd1/1 -> Out1/1

== system gm_rmsNormalization/DUT/BeatAccumulator/AccumulateAdd01 ==
  In1 : Inport
  In2 : Inport  Port=2
  AccumulateAdd01 : Sum  OutDataTypeStr=single  SampleTime=1
  AccumulateAdd01_pd1 : Delay  DelayLength=11
  Out1 : Outport
  wires:
  In1/1 -> AccumulateAdd01/1
  In2/1 -> AccumulateAdd01/2
  AccumulateAdd01/1 -> AccumulateAdd01_pd1/1
  AccumulateAdd01_pd1/1 -> Out1/1

== system gm_rmsNormalization/DUT/BeatAccumulator/AccumulateAdd02 ==
  In1 : Inport
  In2 : Inport  Port=2
  AccumulateAdd02 : Sum  OutDataTypeStr=single  SampleTime=1
  AccumulateAdd02_pd1 : Delay  DelayLength=11
  Out1 : Outport
  wires:
  In1/1 -> AccumulateAdd02/1
  In2/1 -> AccumulateAdd02/2
  AccumulateAdd02/1 -> AccumulateAdd02_pd1/1
  AccumulateAdd02_pd1/1 -> Out1/1

== system gm_rmsNormalization/DUT/BeatAccumulator/AccumulateAdd03 ==
  In1 : Inport
  In2 : Inport  Port=2
  AccumulateAdd03 : Sum  OutDataTypeStr=single  SampleTime=1
  AccumulateAdd03_pd1 : Delay  DelayLength=11
  Out1 : Outport
  wires:
  In1/1 -> AccumulateAdd03/1
  In2/1 -> AccumulateAdd03/2
  AccumulateAdd03/1 -> AccumulateAdd03_pd1/1
  AccumulateAdd03_pd1/1 -> Out1/1

== system gm_rmsNormalization/DUT/BeatAccumulator/AccumulateAdd04 ==
  In1 : Inport
  In2 : Inport  Port=2
  AccumulateAdd04 : Sum  OutDataTypeStr=single  SampleTime=1
  AccumulateAdd04_pd1 : Delay  DelayLength=11
  Out1 : Outport
  wires:
  In1/1 -> AccumulateAdd04/1
  In2/1 -> AccumulateAdd04/2
  AccumulateAdd04/1 -> AccumulateAdd04_pd1/1
  AccumulateAdd04_pd1/1 -> Out1/1

== system gm_rmsNormalization/DUT/BeatAccumulator/AccumulateAdd05 ==
  In1 : Inport
  In2 : Inport  Port=2
  AccumulateAdd05 : Sum  OutDataTypeStr=single  SampleTime=1
  AccumulateAdd05_pd1 : Delay  DelayLength=11
  Out1 : Outport
  wires:
  In1/1 -> AccumulateAdd05/1
  In2/1 -> AccumulateAdd05/2
  AccumulateAdd05/1 -> AccumulateAdd05_pd1/1
  AccumulateAdd05_pd1/1 -> Out1/1

== system gm_rmsNormalization/DUT/BeatAccumulator/AccumulateAdd06 ==
  In1 : Inport
  In2 : Inport  Port=2
  AccumulateAdd06 : Sum  OutDataTypeStr=single  SampleTime=1
  AccumulateAdd06_pd1 : Delay  DelayLength=11
  Out1 : Outport
  wires:
  In1/1 -> AccumulateAdd06/1
  In2/1 -> AccumulateAdd06/2
  AccumulateAdd06/1 -> AccumulateAdd06_pd1/1
  AccumulateAdd06_pd1/1 -> Out1/1

== system gm_rmsNormalization/DUT/BeatAccumulator/AccumulateAdd07 ==
  In1 : Inport
  In2 : Inport  Port=2
  AccumulateAdd07 : Sum  OutDataTypeStr=single  SampleTime=1
  AccumulateAdd07_pd1 : Delay  DelayLength=11
  Out1 : Outport
  wires:
  In1/1 -> AccumulateAdd07/1
  In2/1 -> AccumulateAdd07/2
  AccumulateAdd07/1 -> AccumulateAdd07_pd1/1
  AccumulateAdd07_pd1/1 -> Out1/1

== system gm_rmsNormalization/DUT/BeatAccumulator/AccumulateAdd08 ==
  In1 : Inport
  In2 : Inport  Port=2
  AccumulateAdd08 : Sum  OutDataTypeStr=single  SampleTime=1
  AccumulateAdd08_pd1 : Delay  DelayLength=11
  Out1 : Outport
  wires:
  In1/1 -> AccumulateAdd08/1
  In2/1 -> AccumulateAdd08/2
  AccumulateAdd08/1 -> AccumulateAdd08_pd1/1
  AccumulateAdd08_pd1/1 -> Out1/1

== system gm_rmsNormalization/DUT/BeatAccumulator/AccumulateAdd09 ==
  In1 : Inport
  In2 : Inport  Port=2
  AccumulateAdd09 : Sum  OutDataTypeStr=single  SampleTime=1
  AccumulateAdd09_pd1 : Delay  DelayLength=11
  Out1 : Outport
  wires:
  In1/1 -> AccumulateAdd09/1
  In2/1 -> AccumulateAdd09/2
  AccumulateAdd09/1 -> AccumulateAdd09_pd1/1
  AccumulateAdd09_pd1/1 -> Out1/1

== system gm_rmsNormalization/DUT/BeatAccumulator/AccumulateAdd10 ==
  In1 : Inport
  In2 : Inport  Port=2
  AccumulateAdd10 : Sum  OutDataTypeStr=single  SampleTime=1
  AccumulateAdd10_pd1 : Delay  DelayLength=11
  Out1 : Outport
  wires:
  In1/1 -> AccumulateAdd10/1
  In2/1 -> AccumulateAdd10/2
  AccumulateAdd10/1 -> AccumulateAdd10_pd1/1
  AccumulateAdd10_pd1/1 -> Out1/1

== system gm_rmsNormalization/DUT/BeatAccumulator/Gate00 ==
  In1 : Inport
  In2 : Inport  Port=2
  Gate00 : Product  Inputs=**  OutDataTypeStr=single  SampleTime=1
  Gate00_pd1 : Delay  DelayLength=8
  Out1 : Outport
  wires:
  In1/1 -> Gate00/1
  In2/1 -> Gate00/2
  Gate00/1 -> Gate00_pd1/1
  Gate00_pd1/1 -> Out1/1

== system gm_rmsNormalization/DUT/BeatAccumulator/Gate001 ==
  In1 : Inport
  In2 : Inport  Port=2
  Gate001 : Product  Inputs=**  OutDataTypeStr=single  SampleTime=1
  Gate001_pd1 : Delay  DelayLength=8
  Out1 : Outport
  wires:
  In1/1 -> Gate001/1
  In2/1 -> Gate001/2
  Gate001/1 -> Gate001_pd1/1
  Gate001_pd1/1 -> Out1/1

== system gm_rmsNormalization/DUT/BeatAccumulator/Gate01 ==
  In1 : Inport
  In2 : Inport  Port=2
  Gate01 : Product  Inputs=**  OutDataTypeStr=single  SampleTime=1
  Gate01_pd1 : Delay  DelayLength=8
  Out1 : Outport
  wires:
  In1/1 -> Gate01/1
  In2/1 -> Gate01/2
  Gate01/1 -> Gate01_pd1/1
  Gate01_pd1/1 -> Out1/1

== system gm_rmsNormalization/DUT/BeatAccumulator/Gate011 ==
  In1 : Inport
  In2 : Inport  Port=2
  Gate011 : Product  Inputs=**  OutDataTypeStr=single  SampleTime=1
  Gate011_pd1 : Delay  DelayLength=8
  Out1 : Outport
  wires:
  In1/1 -> Gate011/1
  In2/1 -> Gate011/2
  Gate011/1 -> Gate011_pd1/1
  Gate011_pd1/1 -> Out1/1

== system gm_rmsNormalization/DUT/BeatAccumulator/Gate02 ==
  In1 : Inport
  In2 : Inport  Port=2
  Gate02 : Product  Inputs=**  OutDataTypeStr=single  SampleTime=1
  Gate02_pd1 : Delay  DelayLength=8
  Out1 : Outport
  wires:
  In1/1 -> Gate02/1
  In2/1 -> Gate02/2
  Gate02/1 -> Gate02_pd1/1
  Gate02_pd1/1 -> Out1/1

== system gm_rmsNormalization/DUT/BeatAccumulator/Gate021 ==
  In1 : Inport
  In2 : Inport  Port=2
  Gate021 : Product  Inputs=**  OutDataTypeStr=single  SampleTime=1
  Gate021_pd1 : Delay  DelayLength=8
  Out1 : Outport
  wires:
  In1/1 -> Gate021/1
  In2/1 -> Gate021/2
  Gate021/1 -> Gate021_pd1/1
  Gate021_pd1/1 -> Out1/1

== system gm_rmsNormalization/DUT/BeatAccumulator/Gate03 ==
  In1 : Inport
  In2 : Inport  Port=2
  Gate03 : Product  Inputs=**  OutDataTypeStr=single  SampleTime=1
  Gate03_pd1 : Delay  DelayLength=8
  Out1 : Outport
  wires:
  In1/1 -> Gate03/1
  In2/1 -> Gate03/2
  Gate03/1 -> Gate03_pd1/1
  Gate03_pd1/1 -> Out1/1

== system gm_rmsNormalization/DUT/BeatAccumulator/Gate031 ==
  In1 : Inport
  In2 : Inport  Port=2
  Gate031 : Product  Inputs=**  OutDataTypeStr=single  SampleTime=1
  Gate031_pd1 : Delay  DelayLength=8
  Out1 : Outport
  wires:
  In1/1 -> Gate031/1
  In2/1 -> Gate031/2
  Gate031/1 -> Gate031_pd1/1
  Gate031_pd1/1 -> Out1/1

== system gm_rmsNormalization/DUT/BeatAccumulator/Gate04 ==
  In1 : Inport
  In2 : Inport  Port=2
  Gate04 : Product  Inputs=**  OutDataTypeStr=single  SampleTime=1
  Gate04_pd1 : Delay  DelayLength=8
  Out1 : Outport
  wires:
  In1/1 -> Gate04/1
  In2/1 -> Gate04/2
  Gate04/1 -> Gate04_pd1/1
  Gate04_pd1/1 -> Out1/1

== system gm_rmsNormalization/DUT/BeatAccumulator/Gate041 ==
  In1 : Inport
  In2 : Inport  Port=2
  Gate041 : Product  Inputs=**  OutDataTypeStr=single  SampleTime=1
  Gate041_pd1 : Delay  DelayLength=8
  Out1 : Outport
  wires:
  In1/1 -> Gate041/1
  In2/1 -> Gate041/2
  Gate041/1 -> Gate041_pd1/1
  Gate041_pd1/1 -> Out1/1

== system gm_rmsNormalization/DUT/BeatAccumulator/Gate05 ==
  In1 : Inport
  In2 : Inport  Port=2
  Gate05 : Product  Inputs=**  OutDataTypeStr=single  SampleTime=1
  Gate05_pd1 : Delay  DelayLength=8
  Out1 : Outport
  wires:
  In1/1 -> Gate05/1
  In2/1 -> Gate05/2
  Gate05/1 -> Gate05_pd1/1
  Gate05_pd1/1 -> Out1/1

== system gm_rmsNormalization/DUT/BeatAccumulator/Gate051 ==
  In1 : Inport
  In2 : Inport  Port=2
  Gate051 : Product  Inputs=**  OutDataTypeStr=single  SampleTime=1
  Gate051_pd1 : Delay  DelayLength=8
  Out1 : Outport
  wires:
  In1/1 -> Gate051/1
  In2/1 -> Gate051/2
  Gate051/1 -> Gate051_pd1/1
  Gate051_pd1/1 -> Out1/1

== system gm_rmsNormalization/DUT/BeatAccumulator/Gate06 ==
  In1 : Inport
  In2 : Inport  Port=2
  Gate06 : Product  Inputs=**  OutDataTypeStr=single  SampleTime=1
  Gate06_pd1 : Delay  DelayLength=8
  Out1 : Outport
  wires:
  In1/1 -> Gate06/1
  In2/1 -> Gate06/2
  Gate06/1 -> Gate06_pd1/1
  Gate06_pd1/1 -> Out1/1

== system gm_rmsNormalization/DUT/BeatAccumulator/Gate061 ==
  In1 : Inport
  In2 : Inport  Port=2
  Gate061 : Product  Inputs=**  OutDataTypeStr=single  SampleTime=1
  Gate061_pd1 : Delay  DelayLength=8
  Out1 : Outport
  wires:
  In1/1 -> Gate061/1
  In2/1 -> Gate061/2
  Gate061/1 -> Gate061_pd1/1
  Gate061_pd1/1 -> Out1/1

== system gm_rmsNormalization/DUT/BeatAccumulator/Gate07 ==
  In1 : Inport
  In2 : Inport  Port=2
  Gate07 : Product  Inputs=**  OutDataTypeStr=single  SampleTime=1
  Gate07_pd1 : Delay  DelayLength=8
  Out1 : Outport
  wires:
  In1/1 -> Gate07/1
  In2/1 -> Gate07/2
  Gate07/1 -> Gate07_pd1/1
  Gate07_pd1/1 -> Out1/1

== system gm_rmsNormalization/DUT/BeatAccumulator/Gate071 ==
  In1 : Inport
  In2 : Inport  Port=2
  Gate071 : Product  Inputs=**  OutDataTypeStr=single  SampleTime=1
  Gate071_pd1 : Delay  DelayLength=8
  Out1 : Outport
  wires:
  In1/1 -> Gate071/1
  In2/1 -> Gate071/2
  Gate071/1 -> Gate071_pd1/1
  Gate071_pd1/1 -> Out1/1

== system gm_rmsNormalization/DUT/BeatAccumulator/Gate08 ==
  In1 : Inport
  In2 : Inport  Port=2
  Gate08 : Product  Inputs=**  OutDataTypeStr=single  SampleTime=1
  Gate08_pd1 : Delay  DelayLength=8
  Out1 : Outport
  wires:
  In1/1 -> Gate08/1
  In2/1 -> Gate08/2
  Gate08/1 -> Gate08_pd1/1
  Gate08_pd1/1 -> Out1/1

== system gm_rmsNormalization/DUT/BeatAccumulator/Gate081 ==
  In1 : Inport
  In2 : Inport  Port=2
  Gate081 : Product  Inputs=**  OutDataTypeStr=single  SampleTime=1
  Gate081_pd1 : Delay  DelayLength=8
  Out1 : Outport
  wires:
  In1/1 -> Gate081/1
  In2/1 -> Gate081/2
  Gate081/1 -> Gate081_pd1/1
  Gate081_pd1/1 -> Out1/1

== system gm_rmsNormalization/DUT/BeatAccumulator/Gate09 ==
  In1 : Inport
  In2 : Inport  Port=2
  Gate09 : Product  Inputs=**  OutDataTypeStr=single  SampleTime=1
  Gate09_pd1 : Delay  DelayLength=8
  Out1 : Outport
  wires:
  In1/1 -> Gate09/1
  In2/1 -> Gate09/2
  Gate09/1 -> Gate09_pd1/1
  Gate09_pd1/1 -> Out1/1

== system gm_rmsNormalization/DUT/BeatAccumulator/Gate091 ==
  In1 : Inport
  In2 : Inport  Port=2
  Gate091 : Product  Inputs=**  OutDataTypeStr=single  SampleTime=1
  Gate091_pd1 : Delay  DelayLength=8
  Out1 : Outport
  wires:
  In1/1 -> Gate091/1
  In2/1 -> Gate091/2
  Gate091/1 -> Gate091_pd1/1
  Gate091_pd1/1 -> Out1/1

== system gm_rmsNormalization/DUT/BeatAccumulator/Gate10 ==
  In1 : Inport
  In2 : Inport  Port=2
  Gate10 : Product  Inputs=**  OutDataTypeStr=single  SampleTime=1
  Gate10_pd1 : Delay  DelayLength=8
  Out1 : Outport
  wires:
  In1/1 -> Gate10/1
  In2/1 -> Gate10/2
  Gate10/1 -> Gate10_pd1/1
  Gate10_pd1/1 -> Out1/1

== system gm_rmsNormalization/DUT/BeatAccumulator/Gate101 ==
  In1 : Inport
  In2 : Inport  Port=2
  Gate101 : Product  Inputs=**  OutDataTypeStr=single  SampleTime=1
  Gate101_pd1 : Delay  DelayLength=8
  Out1 : Outport
  wires:
  In1/1 -> Gate101/1
  In2/1 -> Gate101/2
  Gate101/1 -> Gate101_pd1/1
  Gate101_pd1/1 -> Out1/1

== system gm_rmsNormalization/DUT/BeatAccumulator/Sum01 ==
  In1 : Inport
  In2 : Inport  Port=2
  Sum01 : Sum  OutDataTypeStr=single  SampleTime=1
  Sum01_pd1 : Delay  DelayLength=11
  Out1 : Outport
  wires:
  In1/1 -> Sum01/1
  In2/1 -> Sum01/2
  Sum01/1 -> Sum01_pd1/1
  Sum01_pd1/1 -> Out1/1

== system gm_rmsNormalization/DUT/BeatAccumulator/Sum0123 ==
  In1 : Inport
  In2 : Inport  Port=2
  Sum0123 : Sum  OutDataTypeStr=single  SampleTime=1
  Sum0123_pd1 : Delay  DelayLength=11
  Out1 : Outport
  wires:
  In1/1 -> Sum0123/1
  In2/1 -> Sum0123/2
  Sum0123/1 -> Sum0123_pd1/1
  Sum0123_pd1/1 -> Out1/1

== system gm_rmsNormalization/DUT/BeatAccumulator/Sum01234567 ==
  In1 : Inport
  In2 : Inport  Port=2
  Sum01234567 : Sum  OutDataTypeStr=single  SampleTime=1
  Sum01234567_pd1 : Delay  DelayLength=11
  Out1 : Outport
  wires:
  In1/1 -> Sum01234567/1
  In2/1 -> Sum01234567/2
  Sum01234567/1 -> Sum01234567_pd1/1
  Sum01234567_pd1/1 -> Out1/1

== system gm_rmsNormalization/DUT/BeatAccumulator/Sum23 ==
  In1 : Inport
  In2 : Inport  Port=2
  Sum23 : Sum  OutDataTypeStr=single  SampleTime=1
  Sum23_pd1 : Delay  DelayLength=11
  Out1 : Outport
  wires:
  In1/1 -> Sum23/1
  In2/1 -> Sum23/2
  Sum23/1 -> Sum23_pd1/1
  Sum23_pd1/1 -> Out1/1

== system gm_rmsNormalization/DUT/BeatAccumulator/Sum45 ==
  In1 : Inport
  In2 : Inport  Port=2
  Sum45 : Sum  OutDataTypeStr=single  SampleTime=1
  Sum45_pd1 : Delay  DelayLength=11
  Out1 : Outport
  wires:
  In1/1 -> Sum45/1
  In2/1 -> Sum45/2
  Sum45/1 -> Sum45_pd1/1
  Sum45_pd1/1 -> Out1/1

== system gm_rmsNormalization/DUT/BeatAccumulator/Sum4567 ==
  In1 : Inport
  In2 : Inport  Port=2
  Sum4567 : Sum  OutDataTypeStr=single  SampleTime=1
  Sum4567_pd1 : Delay  DelayLength=11
  Out1 : Outport
  wires:
  In1/1 -> Sum4567/1
  In2/1 -> Sum4567/2
  Sum4567/1 -> Sum4567_pd1/1
  Sum4567_pd1/1 -> Out1/1

== system gm_rmsNormalization/DUT/BeatAccumulator/Sum67 ==
  In1 : Inport
  In2 : Inport  Port=2
  Sum67 : Sum  OutDataTypeStr=single  SampleTime=1
  Sum67_pd1 : Delay  DelayLength=11
  Out1 : Outport
  wires:
  In1/1 -> Sum67/1
  In2/1 -> Sum67/2
  Sum67/1 -> Sum67_pd1/1
  Sum67_pd1/1 -> Out1/1

== system gm_rmsNormalization/DUT/BeatAccumulator/Sum89 ==
  In1 : Inport
  In2 : Inport  Port=2
  Sum89 : Sum  OutDataTypeStr=single  SampleTime=1
  Sum89_pd1 : Delay  DelayLength=11
  Out1 : Outport
  wires:
  In1/1 -> Sum89/1
  In2/1 -> Sum89/2
  Sum89/1 -> Sum89_pd1/1
  Sum89_pd1/1 -> Out1/1

== system gm_rmsNormalization/DUT/BeatAccumulator/Sum8910 ==
  In1 : Inport
  In2 : Inport  Port=2
  Sum8910 : Sum  OutDataTypeStr=single  SampleTime=1
  Sum8910_pd1 : Delay  DelayLength=11
  Out1 : Outport
  wires:
  In1/1 -> Sum8910/1
  In2/1 -> Sum8910/2
  Sum8910/1 -> Sum8910_pd1/1
  Sum8910_pd1/1 -> Out1/1

== system gm_rmsNormalization/DUT/BeatAccumulator/SumAll ==
  In1 : Inport
  In2 : Inport  Port=2
  SumAll : Sum  OutDataTypeStr=single  SampleTime=1
  SumAll_pd1 : Delay  DelayLength=11
  Out1 : Outport
  wires:
  In1/1 -> SumAll/1
  In2/1 -> SumAll/2
  SumAll/1 -> SumAll_pd1/1
  SumAll_pd1/1 -> Out1/1

== system gm_rmsNormalization/DUT/BeatReduce/Add01 ==
  In1 : Inport
  In2 : Inport  Port=2
  Add01 : Sum  OutDataTypeStr=single  SampleTime=1
  Add01_pd1 : Delay  DelayLength=11
  Out1 : Outport
  wires:
  In1/1 -> Add01/1
  In2/1 -> Add01/2
  Add01/1 -> Add01_pd1/1
  Add01_pd1/1 -> Out1/1

== system gm_rmsNormalization/DUT/BeatReduce/Add0123 ==
  In1 : Inport
  In2 : Inport  Port=2
  Add0123 : Sum  OutDataTypeStr=single  SampleTime=1
  Add0123_pd1 : Delay  DelayLength=11
  Out1 : Outport
  wires:
  In1/1 -> Add0123/1
  In2/1 -> Add0123/2
  Add0123/1 -> Add0123_pd1/1
  Add0123_pd1/1 -> Out1/1

== system gm_rmsNormalization/DUT/BeatReduce/Add23 ==
  In1 : Inport
  In2 : Inport  Port=2
  Add23 : Sum  OutDataTypeStr=single  SampleTime=1
  Add23_pd1 : Delay  DelayLength=11
  Out1 : Outport
  wires:
  In1/1 -> Add23/1
  In2/1 -> Add23/2
  Add23/1 -> Add23_pd1/1
  Add23_pd1/1 -> Out1/1

== system gm_rmsNormalization/DUT/BeatReduce/Add45 ==
  In1 : Inport
  In2 : Inport  Port=2
  Add45 : Sum  OutDataTypeStr=single  SampleTime=1
  Add45_pd1 : Delay  DelayLength=11
  Out1 : Outport
  wires:
  In1/1 -> Add45/1
  In2/1 -> Add45/2
  Add45/1 -> Add45_pd1/1
  Add45_pd1/1 -> Out1/1

== system gm_rmsNormalization/DUT/BeatReduce/Add4567 ==
  In1 : Inport
  In2 : Inport  Port=2
  Add4567 : Sum  OutDataTypeStr=single  SampleTime=1
  Add4567_pd1 : Delay  DelayLength=11
  Out1 : Outport
  wires:
  In1/1 -> Add4567/1
  In2/1 -> Add4567/2
  Add4567/1 -> Add4567_pd1/1
  Add4567_pd1/1 -> Out1/1

== system gm_rmsNormalization/DUT/BeatReduce/Add67 ==
  In1 : Inport
  In2 : Inport  Port=2
  Add67 : Sum  OutDataTypeStr=single  SampleTime=1
  Add67_pd1 : Delay  DelayLength=11
  Out1 : Outport
  wires:
  In1/1 -> Add67/1
  In2/1 -> Add67/2
  Add67/1 -> Add67_pd1/1
  Add67_pd1/1 -> Out1/1

== system gm_rmsNormalization/DUT/BeatReduce/AddAll ==
  In1 : Inport
  In2 : Inport  Port=2
  AddAll : Sum  OutDataTypeStr=single  SampleTime=1
  AddAll_pd1 : Delay  DelayLength=11
  Out1 : Outport
  wires:
  In1/1 -> AddAll/1
  In2/1 -> AddAll/2
  AddAll/1 -> AddAll_pd1/1
  AddAll_pd1/1 -> Out1/1

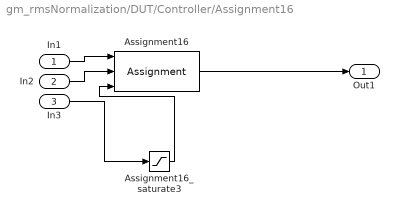
== system gm_rmsNormalization/DUT/Controller/Assignment16 ==
  In1 : Inport
  In2 : Inport  Port=2
  In3 : Inport  Port=3
  Assignment16 : Assignment  IndexOptions=Index vector (port)  Indices=double(-1)  OutputSizes=double(0)
  Assignment16_saturate3 : Saturate  UpperLimit=1536  LowerLimit=1
  Out1 : Outport
  wires:
  In3/1 -> Assignment16_saturate3/1
  Assignment16_saturate3/1 -> Assignment16/3
  In1/1 -> Assignment16/1
  In2/1 -> Assignment16/2
  Assignment16/1 -> Out1/1

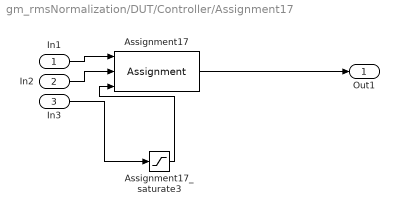
== system gm_rmsNormalization/DUT/Controller/Assignment17 ==
  In1 : Inport
  In2 : Inport  Port=2
  In3 : Inport  Port=3
  Assignment17 : Assignment  IndexOptions=Index vector (port)  Indices=double(-1)  OutputSizes=double(0)
  Assignment17_saturate3 : Saturate  UpperLimit=1536  LowerLimit=1
  Out1 : Outport
  wires:
  In3/1 -> Assignment17_saturate3/1
  Assignment17_saturate3/1 -> Assignment17/3
  In1/1 -> Assignment17/1
  In2/1 -> Assignment17/2
  Assignment17/1 -> Out1/1

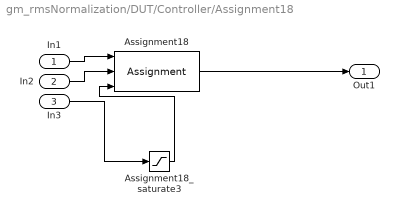
== system gm_rmsNormalization/DUT/Controller/Assignment18 ==
  In1 : Inport
  In2 : Inport  Port=2
  In3 : Inport  Port=3
  Assignment18 : Assignment  IndexOptions=Index vector (port)  Indices=double(-1)  OutputSizes=double(0)
  Assignment18_saturate3 : Saturate  UpperLimit=1536  LowerLimit=1
  Out1 : Outport
  wires:
  In3/1 -> Assignment18_saturate3/1
  Assignment18_saturate3/1 -> Assignment18/3
  In1/1 -> Assignment18/1
  In2/1 -> Assignment18/2
  Assignment18/1 -> Out1/1
